simulink model "Copy_of_test_CSAD"  (R2017a)
settings: Solver=ode45  StartTime=0.0  StopTime=test_time  FixedStep=0.005  RelTol=1e-3  EnableMultiTasking=on
values from neighbouring files (symbols this model uses):
  Tau_test = [0;0;test]    [model_design.m]
settings Model: Creator=mikkelsorensen  LastModifiedBy=ONLyn
settings DataIOCC: LimitDataPoints=on  SaveFormat=Array
settings OptimizationCC: LifeSpan=inf
settings DebuggingCC: SolverPrmCheckMsg=warning  SFUnexpectedBacktrackingDiag=warning  SFNoUnconditionalDefaultTransitionDiag=warning  SFExecutionAtInitializationDiag=none
settings HardwareCC: ProdBitPerPointer=32  ProdBitPerSizeT=32  ProdBitPerPtrDiffT=32  ProdLargestAtomicFloat=None  ProdIntDivRoundTo=Undefined  ProdEndianess=Unspecified  ProdWordSize=32  ProdHWDeviceType=32-bit Generic
settings ModelReferenceCC: PropagateSignalLabelsOutOfModel=off
settings GRTTargetCC: TargetLangStandard=C89/C90 (ANSI)  GeneratePreprocessorConditionals=Disable all
settings ConfigComp: CovMetricSettings=dw  CovHtmlReporting=on  CovSaveCumulativeToWorkspaceVar=on  CovSaveSingleToWorkspaceVar=on  CovExternalEMLEnable=off  CovSFcnEnable=off

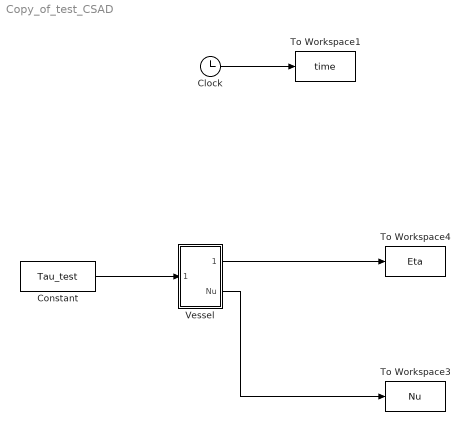
== system Copy_of_test_CSAD ==
  Clock : Clock
  Constant : Constant  Value=Tau_test
  To Workspace1 : ToWorkspace  VariableName=time  SampleTime=-1
  To Workspace3 : ToWorkspace  VariableName=Nu  SampleTime=-1
  To Workspace4 : ToWorkspace  VariableName=Eta  SampleTime=-1
  Vessel : Subsystem
  wires:
  Vessel/1(Eta) -> To Workspace4/1
  Vessel/2(Nu) -> To Workspace3/1
  Clock/1 -> To Workspace1/1
  Constant/1 -> Vessel/1(Tau)

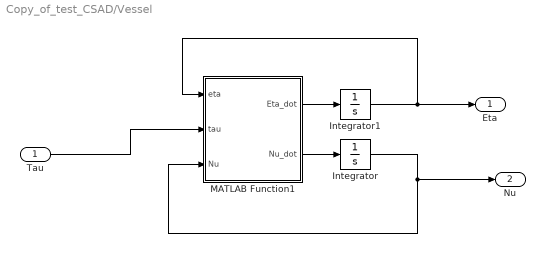
== system Copy_of_test_CSAD/Vessel ==
  Tau : Inport
  Integrator : Integrator  InitialCondition=[0.0 0 0.0]
  Integrator1 : Integrator  InitialCondition=[0 0 0]
  MATLAB Function1 : MATLAB Function  TreatAsAtomicUnit=on
  Eta : Outport
  Nu : Outport  Port=2
  wires:
  Integrator/1 -> Nu/1, MATLAB Function1/3(Nu)
  MATLAB Function1/1(Eta_dot) -> Integrator1/1
  Integrator1/1 -> Eta/1, MATLAB Function1/1(eta)
  MATLAB Function1/2(Nu_dot) -> Integrator/1
  Tau/1 -> MATLAB Function1/2(tau)

== matlab function Copy_of_test_CSAD/Vessel/MATLAB Function1 ==
  data: eta input; tau input; Eta_dot output; Nu input; Nu_dot output
function [Eta_dot,Nu_dot] = Vessel(eta,tau,Nu)

Nu_dot = CSAD_full_old(Nu,tau);

yaw = eta(3);

R =[cos(yaw) -sin(yaw) 0;
            sin(yaw)  cos(yaw) 0;
            0         0        1]; 
Eta_dot = R*Nu;
end
